simulink model "STM32_FIR_test_script_sym"  (R2018a)
settings: Solver=FixedStepAuto  StartTime=0.0  StopTime=10.0  RelTol=1e-3  EnableMultiTasking=on
libraries: stm32f769ilib x2
settings Model: Creator=hpong  LastModifiedBy=hpong
settings OptimizationCC: EnhancedBackFolding=on  PassReuseOutputArgsAs=Individual arguments  MaxStackSize=64  OptimizeBlockOrder=speed  DifferentSizesBufferReuse=on  OptimizationCustomize=off
settings DebuggingCC: ParameterTunabilityLossMsg=error
settings HardwareCC: ProdBitPerPointer=32  ProdBitPerSizeT=32  ProdBitPerPtrDiffT=32  ProdLargestAtomicInteger=Long  ProdLargestAtomicFloat=Double  ProdWordSize=32  ProdHWDeviceType=ARM Compatible->ARM Cortex
settings SFSimCC: MATLABDynamicMemAlloc=off
settings RTWCC: SystemTargetFile=ert.tlc  HardwareBoard=STM32F769I-Discovery  TLCOptions=-aInlineSetEventsForThisBaseRateFcn=TLC_FALSE -aSuppressMultiTaskScheduler=TLC_FALSE -aRateBasedStepFcn=1  TemplateMakefile=ert_default_tmf  GenerateReport=on  Toolchain=GNU Tools for ARM Embedded Processors  IncludeHyperlinkInReport=on  LaunchReport=on  GenerateTraceInfo=on  GenerateTraceReport=on  GenerateTraceReportSl=on  GenerateTraceReportSf=on  GenerateTraceReportEml=on
settings CodeAppCC: ForceParamTrailComments=on  IgnoreCustomStorageClasses=off  OperatorAnnotations=on  SimulinkDataObjDesc=on  SFDataObjDesc=on  InsertBlockDesc=on
settings ERTTargetCC: CodeReplacementLibrary=ARM Cortex-M (CMSIS)  SupportComplex=off

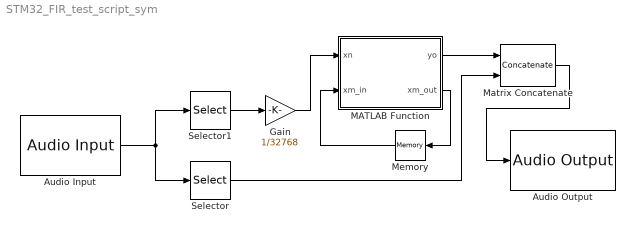
== system STM32_FIR_test_script_sym ==
  Audio Input : stm32f769ilib/Audio Input  InputDevice=LineIn  SamplingFreq=48000  NumCh=2  FrameSize=12
      settings: SourceProductName=Embedded Coder Support Package for STMicroelectronics Discovery Boards  SourceProductBaseCode=STMICRODIS
  Audio Output : stm32f769ilib/Audio Output  OutputDevice=Headphone  SamplingFreq=48000  Volume=65
      settings: SourceProductName=Embedded Coder Support Package for STMicroelectronics Discovery Boards  SourceProductBaseCode=STMICRODIS
  Gain : Gain  Gain=1/32768  OutDataTypeStr=double
  MATLAB Function : MATLAB Function  TreatAsAtomicUnit=on
  Matrix Concatenate : Concatenate  Mode=Multidimensional array  ConcatenateDimension=2
  Memory : Memory  InitialCondition="[0  0  0  0  0  0  0  0  0  0  0  0  0  0  0  0  0  0  0  0  0  0  0  0  0  0  0  0  0  0  0  0  0  0  0  0  0  0  0  0  0  0  0  0  0  0  0  0  0  0  0  0  0  0  0  0  0  0  0  0  0  0  0  0  0  0  0  0  0  0  0  0  0  0  0  0  0  0  0  0  0  0  0  0  0  0  0  0  0  0  ]"  InheritSampleTime=on
  Selector : Selector  NumberOfDimensions=2  InputPortWidth=2  IndexOptions=Select all,Index vector (dialog)  Indices=1,2  OutputSizes=1,1
  Selector1 : Selector  NumberOfDimensions=2  InputPortWidth=2  IndexOptions=Select all,Index vector (dialog)  Indices=1,1  OutputSizes=1,1
  wires:
  Matrix Concatenate/1 -> Audio Output/1
  Audio Input/1 -> Selector1/1, Selector/1
  Selector/1 -> Matrix Concatenate/2
  Selector1/1 -> Gain/1
  MATLAB Function/2(xm_out) -> Memory/1
  Memory/1 -> MATLAB Function/2(xm_in)
  Gain/1 -> MATLAB Function/1(xn)
  MATLAB Function/1(yo) -> Matrix Concatenate/1

== matlab function STM32_FIR_test_script_sym/MATLAB Function ==
  data: xn input; yo output; xm_in input; xm_out output
function [yo, xm_out] = fir_test_sym(xn, xm_in)
b = [0.000000000000000  0.000344388332301  0.000593781079195  0.000648041027613  0.000445668976708  -0.000000000000000  -0.000573654534002  -0.001064568443825  -0.001224479966645  -0.000870953124588  0.000000000000000  0.001148822871272  0.002126699151061  0.002425469036834  0.001703899084196  -0.000000000000000  -0.002179402971244  -0.003968908143450  -0.004453648220912  -0.003080112368334  0.000000000000000  0.003828695228993  0.006885204038667  0.007639273122291  0.005231059848285  -0.000000000000000  -0.006403053722797  -0.011454177756395  -0.012664369033126  -0.008658641008984  0.000000000000000  0.010637147907124  0.019139130184696  0.021353552466227  0.014789178607870  -0.000000000000000  -0.018931847758297  -0.035139742851732  -0.040852871530627  -0.029894735913956  0.000000000000000  0.045867128566198  0.099735326139990  0.150445557587165  0.186587855688577  0.199678576807297  0.186587855688577  0.150445557587165  0.099735326139990  0.045867128566198  0.000000000000000  -0.029894735913956  -0.040852871530627  -0.035139742851732  -0.018931847758297  -0.000000000000000  0.014789178607870  0.021353552466227  0.019139130184696  0.010637147907124  0.000000000000000  -0.008658641008984  -0.012664369033126  -0.011454177756395  -0.006403053722797  -0.000000000000000  0.005231059848285  0.007639273122291  0.006885204038667  0.003828695228993  0.000000000000000  -0.003080112368334  -0.004453648220912  -0.003968908143450  -0.002179402971244  -0.000000000000000  0.001703899084196  0.002425469036834  0.002126699151061  0.001148822871272  0.000000000000000  -0.000870953124588  -0.001224479966645  -0.001064568443825  -0.000573654534002  -0.000000000000000  0.000445668976708  0.000648041027613  0.000593781079195  0.000344388332301  0.000000000000000  ];
nb = length(b);
half_nb = (nb-1)/2;
y=ones(12,1,'double');
xm = xm_in; %4*1
for n=1:12
    y(n) = b(1)* (xn(n)+ xm(nb-1)) + b(half_nb+1)*xm(half_nb);
    for nn=2:half_nb-1
    y(n) = y(n) +  b(nn+1)* (xm(nn) + xm(nb-1-nn)) ; 
    end 
  for i=nb-2:-1:1
     xm(i+1) = xm(i); 
  end
  xm(1) = xn(n);
end
yo = int16(y.*32768);
xm_out = xm;
end
